simulink model "HVDC_VSC_1CPUcore_dcpl"  (Simulink 8.4)
settings: Solver=ode3  SolverMode=SingleTasking  StartTime=0.0  StopTime=70.0  FixedStep=Ts_Power  RelTol=1e-3  AbsTol=1e-2
PreLoadFcn:
  | Ts_Power=50e-6; Ts_Control=1*Ts_Power; init_cosim_IA; startup_transients_hvdc_vsc;
PostLoadFcn:
  | Ts_Power=50e-6; Ts_Control=1*Ts_Power; init_cosim_IA; startup_transients_hvdc_vsc;
InitFcn:
  | Ts_Power=50e-6; Ts_Control=1*Ts_Power; init_cosim_IA; startup_transients_hvdc_vsc;
undefined symbols (not defined in the file): CLARK, D1, Delta, dPref1_2, dPref1_2_rlimit, gcbh, h, intfDelay, level, lib_mesures, magnitude, ResistanceM, rte_drive_private_lib, rte_tsb3level_hiz_rect_cb, sps_rtmsupport, t_deblock_Pref1, t_deblock_Udref2, t_dPref1_2, t_SwitchITMIdc, t_SwitchITMVdc, Ts_intf, TSB3_hiZR
libraries: powerlib x183, spsVIMeasurementModel x102, powerlib_extras x71, powerlib_meascontrol x50, rteventslib x26, op_dpl_lib x20, rtlab x14, sps_avr x6, artemis x1
(part 10 of 13)

== system HVDC_VSC_1CPUcore_dcpl/SS_HVDCStation2_WSCC2/WSCC System 2/Bus_9 230 KV/Three-Phase V-I Measurement3 ==
  Kv : Gain  Gain=Ki  SaturateOnIntegerOverflow=on  OutDataTypeStr=Inherit: Same as input  ParamDataTypeStr=Inherit: Same as input
  Kv1 : Gain  Gain=Kv  SaturateOnIntegerOverflow=on  OutDataTypeStr=Inherit: Same as input  ParamDataTypeStr=Inherit: Same as input
  Mode I : spsVIMeasurementModel/Complex
  Mode V : spsVIMeasurementModel/Complex
  Model : spsVIMeasurementModel/VI_phase  SystemSampleTime=-1
  A : PMIOPort  Port=1  Side=Left
  B : PMIOPort  Port=2  Side=Left
  C : PMIOPort  Port=3  Side=Left
  a : PMIOPort  Port=4  Side=Right
  b : PMIOPort  Port=5  Side=Right
  c : PMIOPort  Port=6  Side=Right
  tag scope: Iabc_30=global, Vabc_30=global
  wires:
  Model/2 -> Kv/1
  Model/1 -> Kv1/1
  Kv/1 -> Mode I/1
  Kv1/1 -> Mode V/1
  Mode I/1 -> [Iabc_30]
  Mode V/1 -> [Vabc_30]
  connections:
  Model/RConn3 -- c/RConn1
  Model/RConn1 -- a/RConn1
  Model/RConn2 -- b/RConn1
  Model/LConn3 -- C/RConn1
  Model/LConn1 -- A/RConn1
  Model/LConn2 -- B/RConn1

== system HVDC_VSC_1CPUcore_dcpl/SS_HVDCStation2_WSCC2/WSCC System 2/Generator BUS1x1/Subsystem1 ==
  In1 : Inport
  In2 : Inport  Port=2
  In3 : Inport  Port=3
  Gain : Gain  Gain=-1  SaturateOnIntegerOverflow=on  OutDataTypeStr=Inherit: Same as input  ParamDataTypeStr=Inherit: Same as input
  Mux : Mux  Inputs=2
  Selector : Selector  InputPortWidth=4  Indices=[4 3]
  Selector1 : Selector  InputPortWidth=4  Indices=[4 3]
  dw_123 : Outport
  T_23 : Outport  Port=2
  wires:
  Selector/1 -> Mux/2
  Mux/1 -> dw_123/1
  In1/1 -> Mux/1
  In2/1 -> Selector/1
  In3/1 -> Selector1/1
  Selector1/1 -> Gain/1
  Gain/1 -> T_23/1

== system HVDC_VSC_1CPUcore_dcpl/SS_HVDCStation2_WSCC2/WSCC System 2/Generator BUS2x1/Subsystem1 ==
  In1 : Inport
  In2 : Inport  Port=2
  In3 : Inport  Port=3
  Gain : Gain  Gain=-1  SaturateOnIntegerOverflow=on  OutDataTypeStr=Inherit: Same as input  ParamDataTypeStr=Inherit: Same as input
  Mux : Mux  Inputs=2
  Selector : Selector  InputPortWidth=4  Indices=[4 3]
  Selector1 : Selector  InputPortWidth=4  Indices=[4 3]
  dw_123 : Outport
  T_23 : Outport  Port=2
  wires:
  Selector/1 -> Mux/2
  Mux/1 -> dw_123/1
  In1/1 -> Mux/1
  In2/1 -> Selector/1
  In3/1 -> Selector1/1
  Selector1/1 -> Gain/1
  Gain/1 -> T_23/1

== system HVDC_VSC_1CPUcore_dcpl/SS_HVDCStation2_WSCC2/WSCC System 2/Generator BUS3x1/Subsystem1 ==
  In1 : Inport
  In2 : Inport  Port=2
  In3 : Inport  Port=3
  Gain : Gain  Gain=-1  SaturateOnIntegerOverflow=on  OutDataTypeStr=Inherit: Same as input  ParamDataTypeStr=Inherit: Same as input
  Mux : Mux  Inputs=2
  Selector : Selector  InputPortWidth=4  Indices=[4 3]
  Selector1 : Selector  InputPortWidth=4  Indices=[4 3]
  dw_123 : Outport
  T_23 : Outport  Port=2
  wires:
  Selector/1 -> Mux/2
  Mux/1 -> dw_123/1
  In1/1 -> Mux/1
  In2/1 -> Selector/1
  In3/1 -> Selector1/1
  Selector1/1 -> Gain/1
  Gain/1 -> T_23/1

== system HVDC_VSC_1CPUcore_dcpl/SM_WSCC1_HVDCStation1/VSC Controller (Station 1)/Discrete VSC Controller (Station 1)/Clark Transformations/CLARK  ==
  note: CLARK transformation
  abc : Inport
  Fcn1 : Fcn  Expr=1/sqrt(3)*(u[2] - u[3])
  Fcn2 : Fcn  Expr=1/3*(2*u[1] - u[2] - u[3])
  Fcn3 : Fcn  Expr=1/3*(u[1] + u[2] + u[3])
  Mux : Mux  Inputs=3
  AB0 : Outport
  wires:
  Fcn2/1 -> Mux/1
  abc/1 -> Fcn1/1, Fcn3/1, Fcn2/1
  Fcn1/1 -> Mux/2
  Fcn3/1 -> Mux/3
  Mux/1 -> AB0/1

== system HVDC_VSC_1CPUcore_dcpl/SM_WSCC1_HVDCStation1/VSC Controller (Station 1)/Discrete VSC Controller (Station 1)/Clark Transformations/CLARK   ==
  note: CLARK transformation
  abc : Inport
  Fcn1 : Fcn  Expr=1/sqrt(3)*(u[2] - u[3])
  Fcn2 : Fcn  Expr=1/3*(2*u[1] - u[2] - u[3])
  Fcn3 : Fcn  Expr=1/3*(u[1] + u[2] + u[3])
  Mux : Mux  Inputs=3
  AB0 : Outport
  wires:
  Mux/1 -> AB0/1
  Fcn3/1 -> Mux/3
  Fcn1/1 -> Mux/2
  abc/1 -> Fcn2/1, Fcn3/1, Fcn1/1
  Fcn2/1 -> Mux/1

== system HVDC_VSC_1CPUcore_dcpl/SM_WSCC1_HVDCStation1/VSC Controller (Station 1)/Discrete VSC Controller (Station 1)/Clark Transformations/CLARK_YD ==
  note: Rotation of pi/6
  note: Rotation of - pi/6
  note: Transformer Connexion:
      | YY = 0
      | YD1 (laging) = 1
      | YD11 (leading)= 2
  note: CLARK transformation
  abc : Inport
  Tr_conx : Inport  Port=2
  CLARK : Subsystem  AncestorBlock=lib_mesures/CLARK  TreatAsAtomicUnit=on
  CLARK_YD1 : Subsystem  AncestorBlock=lib_mesures/CLARK  TreatAsAtomicUnit=on
  CLARK_YD11 : Subsystem  AncestorBlock=lib_mesures/CLARK  TreatAsAtomicUnit=on
  Constant : Constant  Value=2
  Constant1 : Constant  Value=0
  Constant2 : Constant
  Relational Operator1 : RelationalOperator  Operator===  InputSameDT=on
  Relational Operator2 : RelationalOperator  Operator===  InputSameDT=on
  Relational Operator3 : RelationalOperator  Operator===  InputSameDT=on
  Sum : Sum  Inputs=+++  SaturateOnIntegerOverflow=on
  AB0 : Outport
  wires:
  Constant2/1 -> Relational Operator3/2
  Relational Operator2/1 -> CLARK/Enable
  Constant1/1 -> Relational Operator2/2
  CLARK/1(AB0) -> Sum/3
  Sum/1 -> AB0/1
  CLARK_YD1/1(AB0) -> Sum/2
  CLARK_YD11/1(AB0) -> Sum/1
  abc/1 -> CLARK/1(abc), CLARK_YD1/1(abc), CLARK_YD11/1(abc)
  Relational Operator1/1 -> CLARK_YD11/Enable
  Relational Operator3/1 -> CLARK_YD1/Enable
  Tr_conx/1 -> Relational Operator3/1, Relational Operator2/1, Relational Operator1/1
  Constant/1 -> Relational Operator1/2

== system HVDC_VSC_1CPUcore_dcpl/SM_WSCC1_HVDCStation1/VSC Controller (Station 1)/Discrete VSC Controller (Station 1)/Clark Transformations/CLARK_YD  ==
  note: CLARK transformation
  note: Transformer Connexion:
      | YY = 0
      | YD1 (laging) = 1
      | YD11 (leading)= 2
  note: Rotation of - pi/6
  note: Rotation of pi/6
  abc : Inport
  Tr_conx : Inport  Port=2
  CLARK : Subsystem  AncestorBlock=lib_mesures/CLARK  TreatAsAtomicUnit=on
  CLARK_YD1 : Subsystem  AncestorBlock=lib_mesures/CLARK  TreatAsAtomicUnit=on
  CLARK_YD11 : Subsystem  AncestorBlock=lib_mesures/CLARK  TreatAsAtomicUnit=on
  Constant : Constant  Value=2
  Constant1 : Constant  Value=0
  Constant2 : Constant
  Relational Operator1 : RelationalOperator  Operator===  InputSameDT=on
  Relational Operator2 : RelationalOperator  Operator===  InputSameDT=on
  Relational Operator3 : RelationalOperator  Operator===  InputSameDT=on
  Sum : Sum  Inputs=+++  SaturateOnIntegerOverflow=on
  AB0 : Outport
  wires:
  Constant/1 -> Relational Operator1/2
  Tr_conx/1 -> Relational Operator1/1, Relational Operator2/1, Relational Operator3/1
  Relational Operator3/1 -> CLARK_YD1/Enable
  Relational Operator1/1 -> CLARK_YD11/Enable
  abc/1 -> CLARK_YD11/1(abc), CLARK_YD1/1(abc), CLARK/1(abc)
  CLARK_YD11/1(AB0) -> Sum/1
  CLARK_YD1/1(AB0) -> Sum/2
  Sum/1 -> AB0/1
  CLARK/1(AB0) -> Sum/3
  Constant1/1 -> Relational Operator2/2
  Relational Operator2/1 -> CLARK/Enable
  Constant2/1 -> Relational Operator3/2

== system HVDC_VSC_1CPUcore_dcpl/SM_WSCC1_HVDCStation1/VSC Controller (Station 1)/Discrete VSC Controller (Station 1)/DC Voltage Balance Control/Regulator ==
  note: Reset states when enabling
  note: Voltage Sign
  note: Reversed Current Sign
  V_ref_lim_abc : Inport
  Iv_abc : Inport  Port=2
  Udc_0_mean : Inport  Port=3
  Enable : EnablePort  StatesWhenEnabling=reset
  Constant1 : Constant  Value=0
  Constant13 : Constant  Value=Ki_dcvbc
  Constant2 : Constant  Value=0
  Constant3 : Constant  Value=-1
  Constant4 : Constant
  Constant5 : Constant
  Constant6 : Constant  Value=-1
  Constant7 : Constant  Value=0
  Constant8 : Constant  Value=Kp_dcvbc
  "PI_regulator " : Subsystem  mask(PI regulator - type 2){max_i=max_out_dcvbc, min_i=min_out_dcvbc, i_ic=0, max_out=max_out_dcvbc, min_out=min_out_dcvbc, Ts=Ts_Control}
      mask prompts: max_i "Integrator maximum  limit:"; min_i "Integrator minimum  limit:"; i_ic "Integrator initial condition:"; max_out "Output maximum limit:"; min_out "Output minimum limit:"; Ts "Sample time: (s)"
  Product : Product  Inputs=3  SaturateOnIntegerOverflow=on  OutDataTypeStr=Inherit: Same as first input
  Relational Operator : RelationalOperator  Operator=<
  Relational Operator1 : RelationalOperator  Operator=<
  Switch : Switch  Threshold=0.5  SaturateOnIntegerOverflow=on
  Switch1 : Switch  Threshold=0.5  SaturateOnIntegerOverflow=on
  dV_ref_abc_dcvbc : Outport
  wires:
  Switch1/1 -> Product/2
  Constant1/1 -> "PI_regulator "/5(Kf), "PI_regulator "/2(Meas)
  Constant13/1 -> "PI_regulator "/3(Ki)
  Constant8/1 -> "PI_regulator "/4(Kp)
  "PI_regulator "/1(Out) -> Product/3
  Constant2/1 -> Relational Operator/2
  Constant3/1 -> Switch/1
  Constant4/1 -> Switch/3
  Relational Operator/1 -> Switch/2
  Constant5/1 -> Switch1/1
  Constant6/1 -> Switch1/3
  Relational Operator1/1 -> Switch1/2
  Switch/1 -> Product/1
  V_ref_lim_abc/1 -> Relational Operator/1
  Product/1 -> dV_ref_abc_dcvbc/1
  Iv_abc/1 -> Relational Operator1/1
  Udc_0_mean/1 -> "PI_regulator "/1(Ord)
  Constant7/1 -> Relational Operator1/2

== system HVDC_VSC_1CPUcore_dcpl/SM_WSCC1_HVDCStation1/VSC Controller (Station 1)/Discrete VSC Controller (Station 1)/Inner Current Loop/AC_Current_Control ==
  note: Uq
  note: Ud
  note: AC Current Control
  note: d axis
  note: q axis
  Iv_dq : Inport
  Iref_dq : Inport  Port=2
  U_dq : Inport  Port=3
  Freq : Inport  Port=4
  Constant1 : Constant  Value=Kp_accc
  Constant13 : Constant  Value=Ki_accc
  Constant2 : Constant  Value=1.0
  Constant3 : Constant  Value=Kf_accc
  Demux : Demux  Outputs=2
  Demux1 : Demux  Outputs=2
  Demux2 : Demux  Outputs=2
  IC: 1.0 : powerlib_extras/Discrete Measurements/Discrete Variable Frequency Mean value  Finit=60  Fmin=f_min_pll  Vinit=1.0  Ts=Ts_Control
  Mux : Mux  Inputs=2
  "PI_regulator " : Subsystem  mask(PI regulator - type 2){max_i=max_out_accc, min_i=min_out_accc, i_ic=0, max_out=max_out_accc, min_out=min_out_accc, Ts=Ts_Control}
      mask prompts: max_i "Integrator maximum  limit:"; min_i "Integrator minimum  limit:"; i_ic "Integrator initial condition:"; max_out "Output maximum limit:"; min_out "Output minimum limit:"; Ts "Sample time: (s)"
  PI_regulator_2 : Subsystem  mask(PI regulator - type 2){max_i=max_out_accc, min_i=min_out_accc, i_ic=0, max_out=max_out_accc, min_out=min_out_accc, Ts=Ts_Control}
      mask prompts: max_i "Integrator maximum  limit:"; min_i "Integrator minimum  limit:"; i_ic "Integrator initial condition:"; max_out "Output maximum limit:"; min_out "Output minimum limit:"; Ts "Sample time: (s)"
  Product : Product  SaturateOnIntegerOverflow=on  OutDataTypeStr=Inherit: Same as first input
  Product1 : Product  SaturateOnIntegerOverflow=on  OutDataTypeStr=Inherit: Same as first input
  Sum2 : Sum  Inputs=+|-|+  SaturateOnIntegerOverflow=on  InputSameDT=on  OutDataTypeStr=Inherit: Same as first input
  Sum3 : Sum  Inputs=--+  SaturateOnIntegerOverflow=on  InputSameDT=on  OutDataTypeStr=Inherit: Same as first input
  "Variable Frequency Mean value IC:1.0 " : powerlib_extras/Discrete Measurements/Discrete Variable Frequency Mean value  Finit=60  Fmin=f_min_pll  Vinit=1.0  Ts=Ts_Control
  Vref_dq_tmp : Outport
  wires:
  Constant3/1 -> Product1/1, Product/2
  Sum3/1 -> Mux/2
  IC: 1.0/1 -> Sum3/3
  Demux2/2 -> IC: 1.0/2
  Product1/1 -> Sum3/2
  Sum2/1 -> Mux/1
  "Variable Frequency Mean value IC:1.0 "/1 -> Sum2/1
  Freq/1 -> IC: 1.0/1, "Variable Frequency Mean value IC:1.0 "/1
  Demux2/1 -> "Variable Frequency Mean value IC:1.0 "/2
  Product/1 -> Sum2/3
  PI_regulator_2/1(Out) -> Sum3/1
  "PI_regulator "/1(Out) -> Sum2/2
  Iref_dq/1 -> Demux1/1
  Iv_dq/1 -> Demux/1
  Demux1/1 -> "PI_regulator "/1(Ord)  "I_ref_d"
  Demux/1 -> Product1/2, "PI_regulator "/2(Meas)  "Iv_d"
  Constant2/1 -> "PI_regulator "/5(Kf), PI_regulator_2/5(Kf)
  Demux/2 -> Product/1, PI_regulator_2/2(Meas)  "Iv_q"
  Constant13/1 -> "PI_regulator "/3(Ki), PI_regulator_2/3(Ki)
  Mux/1 -> Vref_dq_tmp/1
  Constant1/1 -> "PI_regulator "/4(Kp), PI_regulator_2/4(Kp)
  Demux1/2 -> PI_regulator_2/1(Ord)  "I_ref_q"
  U_dq/1 -> Demux2/1

== system HVDC_VSC_1CPUcore_dcpl/SM_WSCC1_HVDCStation1/VSC Controller (Station 1)/Discrete VSC Controller (Station 1)/Inner Current Loop/Inverse_Clark ==
  note: Inverse CLARK transformation
  AB0 : Inport
  Fcn1 : Fcn  Expr="1/2*(-u[1]  + sqrt(3)*u[2] + 2*u[3])"
  Fcn2 : Fcn  Expr=(u[1] - u[3])
  Fcn3 : Fcn  Expr=1/2*(-u[1] - sqrt(3)*u[2] + 2*u[3])
  Mux : Mux  Inputs=3
  abc : Outport
  wires:
  Fcn2/1 -> Mux/1
  AB0/1 -> Fcn1/1, Fcn3/1, Fcn2/1
  Fcn1/1 -> Mux/2
  Fcn3/1 -> Mux/3
  Mux/1 -> abc/1

== system HVDC_VSC_1CPUcore_dcpl/SM_WSCC1_HVDCStation1/VSC Controller (Station 1)/Discrete VSC Controller (Station 1)/Inner Current Loop/Reference_Voltage_Conditioning ==
  note: Maximum AC Voltage / DC Voltage (pole-neutral)
  note: Voltage Reference Conditioning
  Vref_dq_tmp : Inport
  Udc_meas_mean : Inport  Port=2
  Constant2 : Constant  Value=K_pwm
  Gain1 : Gain  Gain=k_pu2nom_Vdc  SaturateOnIntegerOverflow=on  OutDataTypeStr=Inherit: Same as input  ParamDataTypeStr=Inherit: Same as input
  Product1 : Product  Inputs=**/  SaturateOnIntegerOverflow=on  OutDataTypeStr=Inherit: Same as first input
  Vref_dq : Outport
  wires:
  Gain1/1 -> Product1/2
  Udc_meas_mean/1 -> Gain1/1
  Product1/1 -> Vref_dq/1
  Vref_dq_tmp/1 -> Product1/1
  Constant2/1 -> Product1/3

== system HVDC_VSC_1CPUcore_dcpl/SM_WSCC1_HVDCStation1/VSC Controller (Station 1)/Discrete VSC Controller (Station 1)/Inner Current Loop/Reference_Voltage_Limitation ==
  note: Limitation on a circle of 1 p.u. radius
  note: Reference Voltage Limitation
  note: Not Limited
  note: Limited
  Vref_dq : Inport
  Constant2 : Constant  Value=1.0
  Math Function : Math  Operator=magnitude^2  SaturateOnIntegerOverflow=on
  Math Function1 : Math  Operator=sqrt  SaturateOnIntegerOverflow=on
  Max=inf Min=eps : Saturate  UpperLimit=1e6  LowerLimit=1e-6
  Product : Product  Inputs=/*  SaturateOnIntegerOverflow=on  OutDataTypeStr=Inherit: Same as first input
  Relational Operator1 : RelationalOperator  Operator=<
  Sum : Sum  Inputs=+  SaturateOnIntegerOverflow=on
  Switch : Switch  Threshold=0.5  SaturateOnIntegerOverflow=on
  Vref_lim_dq : Outport
  wires:
  Max=inf Min=eps/1 -> Product/1
  Relational Operator1/1 -> Switch/2
  Math Function1/1 -> Max=inf Min=eps/1, Relational Operator1/1
  Vref_dq/1 -> Math Function/1, Switch/1, Product/2
  Math Function/1 -> Sum/1
  Sum/1 -> Math Function1/1
  Product/1 -> Switch/3
  Switch/1 -> Vref_lim_dq/1
  Constant2/1 -> Relational Operator1/2

== system HVDC_VSC_1CPUcore_dcpl/SM_WSCC1_HVDCStation1/VSC Controller (Station 1)/Discrete VSC Controller (Station 1)/Inner Current Loop/dq0 to abo ==
  note: X0 = X0
  note: dq0 to ab0
  note: Xa = Xd*sin(wt) + Xq*cos(wt)
  note: Xb = -Xd*cos(wt) + Xq*sin(wt)
  dq0 : Inport
  sin_cos : Inport  Port=2
  Demux : Demux  Outputs=2
  Demux1 : Demux  Outputs=3
  Mux : Mux  Inputs=3
  Product{,1..3} (4 alike) : Product  SaturateOnIntegerOverflow=on  InputSameDT=on  OutDataTypeStr=Inherit: Same as first input
  Sum1 : Sum  Inputs=+-  SaturateOnIntegerOverflow=on  InputSameDT=on  OutDataTypeStr=Inherit: Same as first input
  Sum4 : Sum  Inputs=2  SaturateOnIntegerOverflow=on  InputSameDT=on  OutDataTypeStr=Inherit: Same as first input
  ab0 : Outport
  wires:
  dq0/1 -> Demux1/1
  Mux/1 -> ab0/1
  Product3/1 -> Sum1/2
  Product2/1 -> Sum1/1
  Product1/1 -> Sum4/1
  Product/1 -> Sum4/2
  sin_cos/1 -> Demux/1
  Sum4/1 -> Mux/1
  Demux1/1 -> Product1/1, Product3/1
  Demux/1 -> Product1/2, Product2/2
  Demux/2 -> Product/2, Product3/2
  Demux1/2 -> Product/1, Product2/1
  Sum1/1 -> Mux/2
  Demux1/3 -> Mux/3

== system HVDC_VSC_1CPUcore_dcpl/SM_WSCC1_HVDCStation1/VSC Controller (Station 1)/Discrete VSC Controller (Station 1)/Outer Active-Reactive Power and Voltage Loop/Active_Power_Control ==
  note: Active Power Control
  enable_control : Inport
  enable_ramp : Inport  Port=2
  Pref : Inport  Port=3
  dPref : Inport  Port=4
  P_meas : Inport  Port=5
  U_meas : Inport  Port=6
  Udc_meas : Inport  Port=7
  Constant1 : Constant  Value=Udc_max
  Constant11 : Constant  Value=Ki_apc
  Constant12 : Constant  Value=Ramp_apc
  Constant13 : Constant  Value=P_max
  Constant14 : Constant  Value=P_min
  Constant2 : Constant  Value=Udc_min
  Constant25 : Constant  Value=Ki_apc_vco
  Constant3 : Constant  Value=Kp_apc_vco
  DC Voltage Control Override : Subsystem  TreatAsAtomicUnit=on
  Freeze_integrator : Subsystem
  Max=P_max Min=P_min : Saturate  UpperLimit=P_max  LowerLimit=P_min
  Ramping : Subsystem
  Regulator : Subsystem  TreatAsAtomicUnit=on
  Sum1 : Sum  SaturateOnIntegerOverflow=on
  Sum2 : Sum  SaturateOnIntegerOverflow=on
  Pref_apc : Outport
  Pref_ramped : Outport  Port=2
  wires:
  U_meas/1 -> Freeze_integrator/1(U_meas)
  Freeze_integrator/1(Freeze) -> Regulator/6(Freeze)
  Constant14/1 -> Regulator/5(min_out)
  Constant13/1 -> Regulator/4(max_out)
  enable_ramp/1 -> Ramping/1(enable_ramp)
  Pref/1 -> Ramping/2(Pref)
  Constant12/1 -> Ramping/3(ramp_apc)
  P_meas/1 -> Regulator/2(Meas)
  Constant11/1 -> Regulator/3(Ki)
  Sum2/1 -> Regulator/1(Ord), Pref_ramped/1
  dPref/1 -> Sum2/2
  Ramping/1(Pref_ramp) -> Sum2/1
  enable_control/1 -> Regulator/Enable, DC Voltage Control Override/Enable
  Regulator/1(Out) -> Sum1/1
  Sum1/1 -> Max=P_max Min=P_min/1
  DC Voltage Control Override/1(Out) -> Sum1/2
  Constant25/1 -> DC Voltage Control Override/1(Ki_apc_vco)
  Constant1/1 -> DC Voltage Control Override/3(Udc_max)
  Constant2/1 -> DC Voltage Control Override/4(Udc_min)
  Udc_meas/1 -> DC Voltage Control Override/5(Udc_meas)
  Constant3/1 -> DC Voltage Control Override/2(Kp_apc_vco)
  Max=P_max Min=P_min/1 -> Pref_apc/1

== system HVDC_VSC_1CPUcore_dcpl/SM_WSCC1_HVDCStation1/VSC Controller (Station 1)/Discrete VSC Controller (Station 1)/Outer Active-Reactive Power and Voltage Loop/Current_Reference_Calculation ==
  note: Current Reference Calculation
  Pref_apc : Inport
  Qref_rpc : Inport  Port=2
  Uf_meas : Inport  Port=3
  2nd-Order Filter : powerlib_extras/Discrete  Control Blocks/Discrete  2nd-Order Filter  FilterType=Lowpass  Fo=f0_crc  Zeta=1/sqrt(2)  Ts=Ts_Control  Initialize=off  Vac_Init=[0.8 -25 60]  Vdc_Init=-0.4  PlotResponse=off  param1=[1 500 1]
  Constant22 : Constant  Value=lim_d_crc
  Constant23 : Constant  Value=lim_q_crc
  Constant24 : Constant  Value=U_level_crc
  Gain1 : Gain  Gain=-1  SaturateOnIntegerOverflow=on  OutDataTypeStr=Inherit: Same as input  ParamDataTypeStr=Inherit: Same as input
  Gain2 : Gain  Gain=-1  SaturateOnIntegerOverflow=on  OutDataTypeStr=Inherit: Same as input  ParamDataTypeStr=Inherit: Same as input
  MinMax : MinMax  Function=max  Inputs=2  SaturateOnIntegerOverflow=on  InputSameDT=on
  Product : Product  Inputs=*/  SaturateOnIntegerOverflow=on  OutDataTypeStr=Inherit: Same as first input
  Product1 : Product  Inputs=/*  SaturateOnIntegerOverflow=on  OutDataTypeStr=Inherit: Same as first input
  S1 : Subsystem  AncestorBlock=|  mask(Limiter with External Limits){}
      | powerlib_extras/Discrete 
      | Control Blocks/Discrete 12-Pulse
      | HVDC Control /Functions
      | (Discrete)/Current Regulator/S16/S6
      mask Display: disp('      Limiter\n')
  S2 : Subsystem  AncestorBlock=|  mask(Limiter with External Limits){}
      | powerlib_extras/Discrete 
      | Control Blocks/Discrete 12-Pulse
      | HVDC Control /Functions
      | (Discrete)/Current Regulator/S16/S6
      mask Display: disp('      Limiter\n')
  sat : Saturate  UpperLimit=1e6  LowerLimit=1e-6
  Iref_d_crc : Outport
  Iref_q_crc : Outport  Port=2
  wires:
  2nd-Order Filter/1 -> MinMax/2
  S2/1("  ") -> Iref_q_crc/1
  S1/1("  ") -> Iref_d_crc/1
  Uf_meas/1 -> 2nd-Order Filter/1
  Constant24/1 -> MinMax/1
  Pref_apc/1 -> Product/1
  sat/1 -> Product/2, Product1/1
  Qref_rpc/1 -> Product1/2
  Product/1 -> S1/2(In)
  Product1/1 -> S2/2(In)
  Constant22/1 -> Gain1/1, S1/1(MAX)
  Gain1/1 -> S1/3(MIN)
  Constant23/1 -> Gain2/1, S2/1(MAX)
  Gain2/1 -> S2/3(MIN)
  MinMax/1 -> sat/1

== system HVDC_VSC_1CPUcore_dcpl/SM_WSCC1_HVDCStation1/VSC Controller (Station 1)/Discrete VSC Controller (Station 1)/Outer Active-Reactive Power and Voltage Loop/Current_Reference_Limitation ==
  note: DC Voltage Control mode (Active power priority)
  note: Power Control mode (Equal scaling)
  note: Current Reference Limitation
  Iref_d_tmp : Inport  PortDimensions=1
  Iref_q_tmp : Inport  Port=2  PortDimensions=1
  P_control : Inport  Port=3
  Constant25 : Constant  Value=Iref_max
  Double click here for  info : Subsystem
      mask Display: disp('?')
  Math Function1 : Math  Operator=sqrt  SaturateOnIntegerOverflow=on
  Math Function2 : Math  Operator=magnitude^2  SaturateOnIntegerOverflow=on
  Math Function3 : Math  Operator=magnitude^2  SaturateOnIntegerOverflow=on
  Math Function4 : Math  Operator=magnitude^2  SaturateOnIntegerOverflow=on
  Math Function5 : Math  Operator=sqrt  SaturateOnIntegerOverflow=on
  Min:eps Max:inf : Saturate  UpperLimit=1e6  LowerLimit=1e-6
  Mux : Mux  Inputs=2
  Mux1 : Mux  Inputs=2
  Product1 : Product  SaturateOnIntegerOverflow=on  OutDataTypeStr=Inherit: Same as first input
  Product2 : Product  Inputs=*/  SaturateOnIntegerOverflow=on  OutDataTypeStr=Inherit: Same as first input
  Relational Operator1 : RelationalOperator
  Relational Operator3 : RelationalOperator
  Sign : Signum
  Sum : Sum  Inputs=+  SaturateOnIntegerOverflow=on
  Sum2 : Sum  Inputs=-+  SaturateOnIntegerOverflow=on
  Switch1 : Switch  Threshold=0.5  SaturateOnIntegerOverflow=on
  Switch2 : Switch  Threshold=0.5  SaturateOnIntegerOverflow=on
  Switch3 : Switch  Threshold=0.5  SaturateOnIntegerOverflow=on
  Iref_dq : Outport
  wires:
  Sign/1 -> Product1/2
  Math Function5/1 -> Product1/1
  Product1/1 -> Mux1/2
  Sum2/1 -> Math Function5/1
  Math Function4/1 -> Sum2/1
  Math Function3/1 -> Sum2/2
  Mux1/1 -> Switch2/3
  Switch1/1 -> Iref_dq/1
  Switch2/1 -> Switch1/1
  Product2/1 -> Switch2/1
  Min:eps Max:inf/1 -> Product2/2
  Relational Operator1/1 -> Switch1/2
  Constant25/1 -> Relational Operator3/2, Switch3/1, Math Function3/1, Relational Operator1/2
  Math Function1/1 -> Min:eps Max:inf/1, Relational Operator1/1
  Mux/1 -> Product2/1, Math Function2/1, Switch1/3
  Iref_q_tmp/1 -> Sign/1, Mux/2
  Iref_d_tmp/1 -> Relational Operator3/1, Switch3/3, Mux/1
  Sum/1 -> Math Function1/1
  Math Function2/1 -> Sum/1
  P_control/1 -> Switch2/2
  Relational Operator3/1 -> Switch3/2
  Switch3/1 -> Mux1/1, Math Function4/1

== system HVDC_VSC_1CPUcore_dcpl/SM_WSCC1_HVDCStation1/VSC Controller (Station 1)/Discrete VSC Controller (Station 1)/Outer Active-Reactive Power and Voltage Loop/DC_Voltage_Control ==
  note: DC Voltage Control
  note: Reset integrator when enabling
  note: pu DC --> pu AC
  Udref : Inport
  Udc_meas : Inport  Port=2
  Ki_dcvc : Inport  Port=3
  Kp_dcvc : Inport  Port=4
  Enable : EnablePort  StatesWhenEnabling=reset
  Constant1 : Constant  Value=0
  Constant2 : Constant  Value=max_i_dcvc
  Constant3 : Constant  Value=min_i_dcvc
  Constant4 : Constant  Value=max_out_dcvc
  Constant5 : Constant
  Constant6 : Constant  Value=min_out_dcvc
  First-Order_LP f0_Udc IC= k_nom2pu_Vdc : powerlib_extras/Discrete  Control Blocks/Discrete 1st-Order Filter  FilterType=Lowpass  Tc=1/(2*pi*f0_Udc)  Ts=Ts_Control  Initialize=on  Vac_Init=[0 0 60]  Vdc_Init=k_nom2pu_Vdc  PlotResponse=off  param1=[1 600 0.1]
  Gain1 : Gain  Gain=k_nom2pu_Vdc  SaturateOnIntegerOverflow=on  OutDataTypeStr=Inherit: Same as input  ParamDataTypeStr=Inherit: Same as input
  Ic=0 : UnitDelay  SampleTime=Ts_Control
  Kf_dcvc : Constant  Value=1.0
  Logical Operator : Logic  Operator=NOT  Inputs=1  AllPortsSameDT=off
  PI : Subsystem  mask(Integrator  With  External  Dynamic  Limits (Discrete)){i_ic=0, Ts=Ts_Control}
      mask prompts: i_ic "Initial Condition:"; Ts "Sample time: (s)"
      mask Display: disp('Discrete-Time\n(Trapezoidal)\nIntegrator\n ')
  Product2 : Product  SaturateOnIntegerOverflow=on  OutDataTypeStr=Inherit: Same as first input
  Product3 : Product  SaturateOnIntegerOverflow=on  OutDataTypeStr=Inherit: Same as first input
  S6 : Subsystem  AncestorBlock=|  mask(Limiter with External Limits){}
      | powerlib_extras/Discrete 
      | Control Blocks/Discrete 12-Pulse
      | HVDC Control /Functions
      | (Discrete)/Current Regulator/S16/S6
      mask Display: disp('      Limiter\n')
  Sum1 : Sum  Inputs=+-  SaturateOnIntegerOverflow=on
  Sum2 : Sum  SaturateOnIntegerOverflow=on
  Sum3 : Sum  Inputs=|+-  SaturateOnIntegerOverflow=on
  Sum4 : Sum  SaturateOnIntegerOverflow=on
  Iref_d_dcvc : Outport
  wires:
  Product3/1 -> Sum2/1
  Kp_dcvc/1 -> Product3/1
  Logical Operator/1 -> PI/5(Hold), PI/6(Reset)
  Constant5/1 -> Logical Operator/1
  Constant1/1 -> PI/7(Reset Value)
  Constant3/1 -> PI/2(Min)
  Constant2/1 -> PI/1(Max)
  Constant6/1 -> S6/3(MIN)
  Constant4/1 -> S6/1(MAX)
  Sum2/1 -> S6/2(In), Sum3/2
  Sum1/1 -> Product3/2, Sum4/1
  PI/1(Out) -> Sum2/2
  Udc_meas/1 -> First-Order_LP f0_Udc IC= k_nom2pu_Vdc/1
  Ki_dcvc/1 -> PI/4(Ki)
  S6/1("  ") -> Sum3/1, Iref_d_dcvc/1
  Sum4/1 -> PI/3(In)
  Ic=0/1 -> Sum4/2
  Sum3/1 -> Product2/2
  Product2/1 -> Ic=0/1
  Kf_dcvc/1 -> Product2/1
  First-Order_LP f0_Udc IC= k_nom2pu_Vdc/1 -> Sum1/2
  Udref/1 -> Gain1/1
  Gain1/1 -> Sum1/1

== system HVDC_VSC_1CPUcore_dcpl/SM_WSCC1_HVDCStation1/VSC Controller (Station 1)/Discrete VSC Controller (Station 1)/Outer Active-Reactive Power and Voltage Loop/Reactive_Power_Control ==
  note: Reactive Power Control
  enable_control : Inport
  Qref : Inport  Port=2
  Q_meas : Inport  Port=3
  U_meas : Inport  Port=4
  AC Voltage Control Override : Subsystem  TreatAsAtomicUnit=on
  Constant1 : Constant  Value=U_max
  Constant2 : Constant  Value=U_min
  Constant25 : Constant  Value=Ki_rpc_vco
  Constant3 : Constant  Value=Kp_rpc_vco
  Constant4 : Constant  Value=Ki_rpc
  Constant5 : Constant  Value=Q_max
  Constant6 : Constant  Value=Q_min
  Freeze_integrator : Subsystem
  Max=Q_max Min=Q_min : Saturate  UpperLimit=Q_max  LowerLimit=Q_min
  Regulator : Subsystem  TreatAsAtomicUnit=on
  Sum2 : Sum  SaturateOnIntegerOverflow=on
  Qref_rpc : Outport
  wires:
  Sum2/1 -> Max=Q_max Min=Q_min/1
  Regulator/1(Out) -> Sum2/1
  Qref/1 -> Regulator/1(Ord)
  Constant5/1 -> Regulator/4(max_out)
  Constant6/1 -> Regulator/5(min_out)
  Constant4/1 -> Regulator/3(Ki)
  Q_meas/1 -> Regulator/2(Meas)
  U_meas/1 -> AC Voltage Control Override/5(U_meas), Freeze_integrator/1(U_meas)
  enable_control/1 -> Regulator/Enable, AC Voltage Control Override/Enable
  Constant25/1 -> AC Voltage Control Override/1(Ki_rpc_vco)
  Constant3/1 -> AC Voltage Control Override/2(Kp_rpc_vco)
  Constant1/1 -> AC Voltage Control Override/3(U_max)
  Constant2/1 -> AC Voltage Control Override/4(U_min)
  AC Voltage Control Override/1(Out) -> Sum2/2
  Max=Q_max Min=Q_min/1 -> Qref_rpc/1
  Freeze_integrator/1(Freeze) -> Regulator/6(freeze)

== system HVDC_VSC_1CPUcore_dcpl/SM_WSCC1_HVDCStation1/VSC Controller (Station 1)/Discrete VSC Controller (Station 1)/PLL/ab0->dq0  ==
  note: Xq = Xa*cos(wt) + Xb*sin(wt)
  note: Xd = Xa*sin(wt) - Xb*cos(wt)
  note: Alpha-Beta-zero to dq0
  note: X0 = X0
  ab0 : Inport
  sin_cos : Inport  Port=2
  Demux : Demux  Outputs=2
  Demux1 : Demux  Outputs=3
  Mux : Mux  Inputs=3
  Product{,1..3} (4 alike) : Product  SaturateOnIntegerOverflow=on  InputSameDT=on  OutDataTypeStr=Inherit: Same as first input
  Sum1 : Sum  Inputs=+-  SaturateOnIntegerOverflow=on  InputSameDT=on  OutDataTypeStr=Inherit: Same as first input
  Sum4 : Sum  Inputs=2  SaturateOnIntegerOverflow=on  InputSameDT=on  OutDataTypeStr=Inherit: Same as first input
  dq0 : Outport
  wires:
  Sum4/1 -> Mux/2
  Sum1/1 -> Mux/1
  sin_cos/1 -> Demux/1
  Demux/2 -> Product/2, Product3/2
  Demux1/1 -> Product/1, Product2/1
  Product/1 -> Sum4/2
  Demux/1 -> Product2/2, Product1/2
  Demux1/2 -> Product1/1, Product3/1
  Product1/1 -> Sum4/1
  Product2/1 -> Sum1/1
  Product3/1 -> Sum1/2
  Mux/1 -> dq0/1
  ab0/1 -> Demux1/1
  Demux1/3 -> Mux/3

== system HVDC_VSC_1CPUcore_dcpl/SM_WSCC1_HVDCStation1/VSC Controller (Station 1)/Discrete VSC Controller (Station 1)/Signal Calculations/Active_Power ==
  note: Active Power Calculation
  U_AB : Inport
  I_AB : Inport  Port=2
  Demux : Demux  Outputs=2
  Demux1 : Demux  Outputs=2
  Product : Product  SaturateOnIntegerOverflow=on  OutDataTypeStr=Inherit: Same as first input
  Product1 : Product  SaturateOnIntegerOverflow=on  OutDataTypeStr=Inherit: Same as first input
  Sum : Sum  SaturateOnIntegerOverflow=on
  Ppcc : Outport
  wires:
  U_AB/1 -> Demux/1
  I_AB/1 -> Demux1/1
  Demux/1 -> Product/1
  Demux1/1 -> Product/2
  Demux/2 -> Product1/1
  Demux1/2 -> Product1/2
  Product/1 -> Sum/1
  Product1/1 -> Sum/2
  Sum/1 -> Ppcc/1

== system HVDC_VSC_1CPUcore_dcpl/SM_WSCC1_HVDCStation1/VSC Controller (Station 1)/Discrete VSC Controller (Station 1)/Signal Calculations/DC_Current ==
  note: DC Current Calculation
  Idc_p : Inport
  Idc_n : Inport  Port=2
  Gain : Gain  Gain=0.5  SaturateOnIntegerOverflow=on  OutDataTypeStr=Inherit: Same as input  ParamDataTypeStr=Inherit: Same as input
  Sum : Sum  Inputs=+-  SaturateOnIntegerOverflow=on
  Idc_meas : Outport
  wires:
  Gain/1 -> Idc_meas/1
  Sum/1 -> Gain/1
  Idc_n/1 -> Sum/2
  Idc_p/1 -> Sum/1

== system HVDC_VSC_1CPUcore_dcpl/SM_WSCC1_HVDCStation1/VSC Controller (Station 1)/Discrete VSC Controller (Station 1)/Signal Calculations/DC_Voltage ==
  note: DC Voltage Calculation
  Udc_p : Inport
  Udc_n : Inport  Port=2
  Gain : Gain  Gain=0.5  SaturateOnIntegerOverflow=on  OutDataTypeStr=Inherit: Same as input  ParamDataTypeStr=Inherit: Same as input
  Sum : Sum  Inputs=+-  SaturateOnIntegerOverflow=on
  Udc_meas : Outport
  wires:
  Udc_p/1 -> Sum/1
  Sum/1 -> Gain/1
  Gain/1 -> Udc_meas/1
  Udc_n/1 -> Sum/2

== system HVDC_VSC_1CPUcore_dcpl/SM_WSCC1_HVDCStation1/VSC Controller (Station 1)/Discrete VSC Controller (Station 1)/Signal Calculations/Filter_Bus_Voltage ==
  note: Filter Bus Voltage Calculation
  Uf_AB : Inport
  Math Function : Math  Operator=magnitude^2  SaturateOnIntegerOverflow=on
  Math Function1 : Math  Operator=sqrt  SaturateOnIntegerOverflow=on
  Sum : Sum  Inputs=+  SaturateOnIntegerOverflow=on
  Uf_meas : Outport
  wires:
  Math Function1/1 -> Uf_meas/1
  Sum/1 -> Math Function1/1
  Math Function/1 -> Sum/1
  Uf_AB/1 -> Math Function/1

== system HVDC_VSC_1CPUcore_dcpl/SM_WSCC1_HVDCStation1/VSC Controller (Station 1)/Discrete VSC Controller (Station 1)/Signal Calculations/Modulation_Index ==
  note: Modulation Index Calculation
  Vref_lim_AB : Inport
  Udc_meas : Inport  Port=2
  Gain1 : Gain  Gain=k_pu2nom_Vdc  SaturateOnIntegerOverflow=on  OutDataTypeStr=Inherit: Same as input  ParamDataTypeStr=Inherit: Same as input
  MAX:10 MIN: 0 : Saturate  UpperLimit=10  LowerLimit=0
  Math Function1 : Math  Operator=magnitude^2  SaturateOnIntegerOverflow=on
  Math Function2 : Math  Operator=sqrt  SaturateOnIntegerOverflow=on
  Product : Product  Inputs=*/  SaturateOnIntegerOverflow=on  OutDataTypeStr=Inherit: Same as first input
  Saturation : Saturate  UpperLimit=1e6  LowerLimit=1e-6
  Sum : Sum  Inputs=+  SaturateOnIntegerOverflow=on
  Mod_index : Outport
  wires:
  Gain1/1 -> Saturation/1
  MAX:10 MIN: 0/1 -> Mod_index/1
  Saturation/1 -> Product/2
  Product/1 -> MAX:10 MIN: 0/1
  Udc_meas/1 -> Gain1/1
  Sum/1 -> Math Function2/1
  Math Function1/1 -> Sum/1
  Math Function2/1 -> Product/1
  Vref_lim_AB/1 -> Math Function1/1

== system HVDC_VSC_1CPUcore_dcpl/SM_WSCC1_HVDCStation1/VSC Controller (Station 1)/Discrete VSC Controller (Station 1)/Signal Calculations/PCC_Voltage ==
  note: Active Power Calculation
  U_AB : Inport
  Math Function : Math  Operator=magnitude^2  SaturateOnIntegerOverflow=on
  Math Function1 : Math  Operator=sqrt  SaturateOnIntegerOverflow=on
  Sum : Sum  Inputs=+  SaturateOnIntegerOverflow=on
  Upcc : Outport
  wires:
  U_AB/1 -> Math Function/1
  Math Function/1 -> Sum/1
  Sum/1 -> Math Function1/1
  Math Function1/1 -> Upcc/1

== system HVDC_VSC_1CPUcore_dcpl/SM_WSCC1_HVDCStation1/VSC Controller (Station 1)/Discrete VSC Controller (Station 1)/Signal Calculations/Reactive_Power ==
  note: Reactive Power Calculation
  U_AB : Inport
  I_AB : Inport  Port=2
  Demux : Demux  Outputs=2
  Demux1 : Demux  Outputs=2
  Product : Product  SaturateOnIntegerOverflow=on  OutDataTypeStr=Inherit: Same as first input
  Product1 : Product  SaturateOnIntegerOverflow=on  OutDataTypeStr=Inherit: Same as first input
  Sum : Sum  Inputs=+-  SaturateOnIntegerOverflow=on
  Qpcc : Outport
  wires:
  Sum/1 -> Qpcc/1
  Product1/1 -> Sum/2
  Product/1 -> Sum/1
  I_AB/1 -> Demux1/1
  U_AB/1 -> Demux/1
  Demux/2 -> Product/2
  Demux1/1 -> Product/1
  Demux/1 -> Product1/1
  Demux1/2 -> Product1/2

== system HVDC_VSC_1CPUcore_dcpl/SM_WSCC1_HVDCStation1/VSC Controller (Station 1)/Discrete VSC Controller (Station 1)/dq  Transformations/ab0_to_dq0 ==
  note: X0 = X0
  note: Alpha-Beta-zero to dq0
  note: Xd = Xa*sin(wt) - Xb*cos(wt)
  note: Xq = Xa*cos(wt) + Xb*sin(wt)
  ab0 : Inport
  sin_cos : Inport  Port=2
  Demux : Demux  Outputs=2
  Demux1 : Demux  Outputs=3
  Gain3 : Gain  Gain=-1  SaturateOnIntegerOverflow=on  OutDataTypeStr=Inherit: Same as input  ParamDataTypeStr=Inherit: Same as input
  Mux : Mux  Inputs=3
  Product{,1..3} (4 alike) : Product  SaturateOnIntegerOverflow=on  InputSameDT=on  OutDataTypeStr=Inherit: Same as first input
  Sum1 : Sum  Inputs=2  SaturateOnIntegerOverflow=on  InputSameDT=on  OutDataTypeStr=Inherit: Same as first input
  Sum4 : Sum  Inputs=2  SaturateOnIntegerOverflow=on  InputSameDT=on  OutDataTypeStr=Inherit: Same as first input
  dq0 : Outport
  wires:
  Demux1/3 -> Mux/3
  ab0/1 -> Demux1/1
  Mux/1 -> dq0/1
  Product3/1 -> Sum1/2
  Product2/1 -> Sum1/1
  Product1/1 -> Sum4/1
  Demux1/2 -> Product3/1, Product1/1
  Demux/1 -> Product1/2, Product2/2
  Product/1 -> Sum4/2
  Demux1/1 -> Product2/1, Product/1
  Demux/2 -> Product/2, Gain3/1
  sin_cos/1 -> Demux/1
  Sum1/1 -> Mux/1
  Gain3/1 -> Product3/2
  Sum4/1 -> Mux/2

== system HVDC_VSC_1CPUcore_dcpl/SM_WSCC1_HVDCStation1/VSC Controller (Station 1)/Discrete VSC Controller (Station 1)/dq  Transformations/ab0_to_dq0    ==
  note: Xq = Xa*cos(wt) + Xb*sin(wt)
  note: Xd = Xa*sin(wt) - Xb*cos(wt)
  note: Alpha-Beta-zero to dq0
  note: X0 = X0
  ab0 : Inport
  sin_cos : Inport  Port=2
  Demux : Demux  Outputs=2
  Demux1 : Demux  Outputs=3
  Gain3 : Gain  Gain=-1  SaturateOnIntegerOverflow=on  OutDataTypeStr=Inherit: Same as input  ParamDataTypeStr=Inherit: Same as input
  Mux : Mux  Inputs=3
  Product{,1..3} (4 alike) : Product  SaturateOnIntegerOverflow=on  InputSameDT=on  OutDataTypeStr=Inherit: Same as first input
  Sum1 : Sum  Inputs=2  SaturateOnIntegerOverflow=on  InputSameDT=on  OutDataTypeStr=Inherit: Same as first input
  Sum4 : Sum  Inputs=2  SaturateOnIntegerOverflow=on  InputSameDT=on  OutDataTypeStr=Inherit: Same as first input
  dq0 : Outport
  wires:
  Sum4/1 -> Mux/2
  Gain3/1 -> Product3/2
  Sum1/1 -> Mux/1
  sin_cos/1 -> Demux/1
  Demux/2 -> Gain3/1, Product/2
  Demux1/1 -> Product/1, Product2/1
  Product/1 -> Sum4/2
  Demux/1 -> Product2/2, Product1/2
  Demux1/2 -> Product1/1, Product3/1
  Product1/1 -> Sum4/1
  Product2/1 -> Sum1/1
  Product3/1 -> Sum1/2
  Mux/1 -> dq0/1
  ab0/1 -> Demux1/1
  Demux1/3 -> Mux/3

== system HVDC_VSC_1CPUcore_dcpl/SS_HVDCStation2_WSCC2/VSC Controller (Station 2)/Discrete VSC Controller (Station 2)/Clark Transformations/CLARK  ==
  note: CLARK transformation
  abc : Inport
  Fcn1 : Fcn  Expr=1/sqrt(3)*(u[2] - u[3])
  Fcn2 : Fcn  Expr=1/3*(2*u[1] - u[2] - u[3])
  Fcn3 : Fcn  Expr=1/3*(u[1] + u[2] + u[3])
  Mux : Mux  Inputs=3
  AB0 : Outport
  wires:
  Fcn2/1 -> Mux/1
  abc/1 -> Fcn1/1, Fcn3/1, Fcn2/1
  Fcn1/1 -> Mux/2
  Fcn3/1 -> Mux/3
  Mux/1 -> AB0/1

== system HVDC_VSC_1CPUcore_dcpl/SS_HVDCStation2_WSCC2/VSC Controller (Station 2)/Discrete VSC Controller (Station 2)/Clark Transformations/CLARK   ==
  note: CLARK transformation
  abc : Inport
  Fcn1 : Fcn  Expr=1/sqrt(3)*(u[2] - u[3])
  Fcn2 : Fcn  Expr=1/3*(2*u[1] - u[2] - u[3])
  Fcn3 : Fcn  Expr=1/3*(u[1] + u[2] + u[3])
  Mux : Mux  Inputs=3
  AB0 : Outport
  wires:
  Mux/1 -> AB0/1
  Fcn3/1 -> Mux/3
  Fcn1/1 -> Mux/2
  abc/1 -> Fcn2/1, Fcn3/1, Fcn1/1
  Fcn2/1 -> Mux/1

== system HVDC_VSC_1CPUcore_dcpl/SS_HVDCStation2_WSCC2/VSC Controller (Station 2)/Discrete VSC Controller (Station 2)/Clark Transformations/CLARK_YD ==
  note: Rotation of pi/6
  note: Rotation of - pi/6
  note: Transformer Connexion:
      | YY = 0
      | YD1 (laging) = 1
      | YD11 (leading)= 2
  note: CLARK transformation
  abc : Inport
  Tr_conx : Inport  Port=2
  CLARK : Subsystem  AncestorBlock=lib_mesures/CLARK  TreatAsAtomicUnit=on
  CLARK_YD1 : Subsystem  AncestorBlock=lib_mesures/CLARK  TreatAsAtomicUnit=on
  CLARK_YD11 : Subsystem  AncestorBlock=lib_mesures/CLARK  TreatAsAtomicUnit=on
  Constant : Constant  Value=2
  Constant1 : Constant  Value=0
  Constant2 : Constant
  Relational Operator1 : RelationalOperator  Operator===  InputSameDT=on
  Relational Operator2 : RelationalOperator  Operator===  InputSameDT=on
  Relational Operator3 : RelationalOperator  Operator===  InputSameDT=on
  Sum : Sum  Inputs=+++  SaturateOnIntegerOverflow=on
  AB0 : Outport
  wires:
  Constant2/1 -> Relational Operator3/2
  Relational Operator2/1 -> CLARK/Enable
  Constant1/1 -> Relational Operator2/2
  CLARK/1(AB0) -> Sum/3
  Sum/1 -> AB0/1
  CLARK_YD1/1(AB0) -> Sum/2
  CLARK_YD11/1(AB0) -> Sum/1
  abc/1 -> CLARK/1(abc), CLARK_YD1/1(abc), CLARK_YD11/1(abc)
  Relational Operator1/1 -> CLARK_YD11/Enable
  Relational Operator3/1 -> CLARK_YD1/Enable
  Tr_conx/1 -> Relational Operator3/1, Relational Operator2/1, Relational Operator1/1
  Constant/1 -> Relational Operator1/2

== system HVDC_VSC_1CPUcore_dcpl/SS_HVDCStation2_WSCC2/VSC Controller (Station 2)/Discrete VSC Controller (Station 2)/Clark Transformations/CLARK_YD  ==
  note: CLARK transformation
  note: Transformer Connexion:
      | YY = 0
      | YD1 (laging) = 1
      | YD11 (leading)= 2
  note: Rotation of - pi/6
  note: Rotation of pi/6
  abc : Inport
  Tr_conx : Inport  Port=2
  CLARK : Subsystem  AncestorBlock=lib_mesures/CLARK  TreatAsAtomicUnit=on
  CLARK_YD1 : Subsystem  AncestorBlock=lib_mesures/CLARK  TreatAsAtomicUnit=on
  CLARK_YD11 : Subsystem  AncestorBlock=lib_mesures/CLARK  TreatAsAtomicUnit=on
  Constant : Constant  Value=2
  Constant1 : Constant  Value=0
  Constant2 : Constant
  Relational Operator1 : RelationalOperator  Operator===  InputSameDT=on
  Relational Operator2 : RelationalOperator  Operator===  InputSameDT=on
  Relational Operator3 : RelationalOperator  Operator===  InputSameDT=on
  Sum : Sum  Inputs=+++  SaturateOnIntegerOverflow=on
  AB0 : Outport
  wires:
  Constant/1 -> Relational Operator1/2
  Tr_conx/1 -> Relational Operator1/1, Relational Operator2/1, Relational Operator3/1
  Relational Operator3/1 -> CLARK_YD1/Enable
  Relational Operator1/1 -> CLARK_YD11/Enable
  abc/1 -> CLARK_YD11/1(abc), CLARK_YD1/1(abc), CLARK/1(abc)
  CLARK_YD11/1(AB0) -> Sum/1
  CLARK_YD1/1(AB0) -> Sum/2
  Sum/1 -> AB0/1
  CLARK/1(AB0) -> Sum/3
  Constant1/1 -> Relational Operator2/2
  Relational Operator2/1 -> CLARK/Enable
  Constant2/1 -> Relational Operator3/2

== system HVDC_VSC_1CPUcore_dcpl/SS_HVDCStation2_WSCC2/VSC Controller (Station 2)/Discrete VSC Controller (Station 2)/DC Voltage Balance Control/Regulator ==
  note: Reset states when enabling
  note: Voltage Sign
  note: Reversed Current Sign
  V_ref_lim_abc : Inport
  Iv_abc : Inport  Port=2
  Udc_0_mean : Inport  Port=3
  Enable : EnablePort  StatesWhenEnabling=reset
  Constant1 : Constant  Value=0
  Constant13 : Constant  Value=Ki_dcvbc
  Constant2 : Constant  Value=0
  Constant3 : Constant  Value=-1
  Constant4 : Constant
  Constant5 : Constant
  Constant6 : Constant  Value=-1
  Constant7 : Constant  Value=0
  Constant8 : Constant  Value=Kp_dcvbc
  "PI_regulator " : Subsystem  mask(PI regulator - type 2){max_i=max_out_dcvbc, min_i=min_out_dcvbc, i_ic=0, max_out=max_out_dcvbc, min_out=min_out_dcvbc, Ts=Ts_Control}
      mask prompts: max_i "Integrator maximum  limit:"; min_i "Integrator minimum  limit:"; i_ic "Integrator initial condition:"; max_out "Output maximum limit:"; min_out "Output minimum limit:"; Ts "Sample time: (s)"
  Product : Product  Inputs=3  SaturateOnIntegerOverflow=on  OutDataTypeStr=Inherit: Same as first input
  Relational Operator : RelationalOperator  Operator=<
  Relational Operator1 : RelationalOperator  Operator=<
  Switch : Switch  Threshold=0.5  SaturateOnIntegerOverflow=on
  Switch1 : Switch  Threshold=0.5  SaturateOnIntegerOverflow=on
  dV_ref_abc_dcvbc : Outport
  wires:
  Switch1/1 -> Product/2
  Constant1/1 -> "PI_regulator "/5(Kf), "PI_regulator "/2(Meas)
  Constant13/1 -> "PI_regulator "/3(Ki)
  Constant8/1 -> "PI_regulator "/4(Kp)
  "PI_regulator "/1(Out) -> Product/3
  Constant2/1 -> Relational Operator/2
  Constant3/1 -> Switch/1
  Constant4/1 -> Switch/3
  Relational Operator/1 -> Switch/2
  Constant5/1 -> Switch1/1
  Constant6/1 -> Switch1/3
  Relational Operator1/1 -> Switch1/2
  Switch/1 -> Product/1
  V_ref_lim_abc/1 -> Relational Operator/1
  Product/1 -> dV_ref_abc_dcvbc/1
  Iv_abc/1 -> Relational Operator1/1
  Udc_0_mean/1 -> "PI_regulator "/1(Ord)
  Constant7/1 -> Relational Operator1/2

== system HVDC_VSC_1CPUcore_dcpl/SS_HVDCStation2_WSCC2/VSC Controller (Station 2)/Discrete VSC Controller (Station 2)/Inner Current Loop/AC_Current_Control ==
  note: Uq
  note: Ud
  note: AC Current Control
  note: d axis
  note: q axis
  Iv_dq : Inport
  Iref_dq : Inport  Port=2
  U_dq : Inport  Port=3
  Freq : Inport  Port=4
  Constant1 : Constant  Value=Kp_accc
  Constant13 : Constant  Value=Ki_accc
  Constant2 : Constant  Value=1.0
  Constant3 : Constant  Value=Kf_accc
  Demux : Demux  Outputs=2
  Demux1 : Demux  Outputs=2
  Demux2 : Demux  Outputs=2
  IC: 1.0 : powerlib_extras/Discrete Measurements/Discrete Variable Frequency Mean value  Finit=50  Fmin=f_min_pll  Vinit=1.0  Ts=Ts_Control
  Mux : Mux  Inputs=2
  "PI_regulator " : Subsystem  mask(PI regulator - type 2){max_i=max_out_accc, min_i=min_out_accc, i_ic=0, max_out=max_out_accc, min_out=min_out_accc, Ts=Ts_Control}
      mask prompts: max_i "Integrator maximum  limit:"; min_i "Integrator minimum  limit:"; i_ic "Integrator initial condition:"; max_out "Output maximum limit:"; min_out "Output minimum limit:"; Ts "Sample time: (s)"
  PI_regulator_2 : Subsystem  mask(PI regulator - type 2){max_i=max_out_accc, min_i=min_out_accc, i_ic=0, max_out=max_out_accc, min_out=min_out_accc, Ts=Ts_Control}
      mask prompts: max_i "Integrator maximum  limit:"; min_i "Integrator minimum  limit:"; i_ic "Integrator initial condition:"; max_out "Output maximum limit:"; min_out "Output minimum limit:"; Ts "Sample time: (s)"
  Product : Product  SaturateOnIntegerOverflow=on  OutDataTypeStr=Inherit: Same as first input
  Product1 : Product  SaturateOnIntegerOverflow=on  OutDataTypeStr=Inherit: Same as first input
  Sum2 : Sum  Inputs=+|-|+  SaturateOnIntegerOverflow=on  InputSameDT=on  OutDataTypeStr=Inherit: Same as first input
  Sum3 : Sum  Inputs=--+  SaturateOnIntegerOverflow=on  InputSameDT=on  OutDataTypeStr=Inherit: Same as first input
  "Variable Frequency Mean value IC:1.0 " : powerlib_extras/Discrete Measurements/Discrete Variable Frequency Mean value  Finit=50  Fmin=f_min_pll  Vinit=1.0  Ts=Ts_Control
  Vref_dq_tmp : Outport
  wires:
  Constant3/1 -> Product1/1, Product/2
  Sum3/1 -> Mux/2
  IC: 1.0/1 -> Sum3/3
  Demux2/2 -> IC: 1.0/2
  Product1/1 -> Sum3/2
  Sum2/1 -> Mux/1
  "Variable Frequency Mean value IC:1.0 "/1 -> Sum2/1
  Freq/1 -> IC: 1.0/1, "Variable Frequency Mean value IC:1.0 "/1
  Demux2/1 -> "Variable Frequency Mean value IC:1.0 "/2
  Product/1 -> Sum2/3
  PI_regulator_2/1(Out) -> Sum3/1
  "PI_regulator "/1(Out) -> Sum2/2
  Iref_dq/1 -> Demux1/1
  Iv_dq/1 -> Demux/1
  Demux1/1 -> "PI_regulator "/1(Ord)  "I_ref_d"
  Demux/1 -> Product1/2, "PI_regulator "/2(Meas)  "Iv_d"
  Constant2/1 -> "PI_regulator "/5(Kf), PI_regulator_2/5(Kf)
  Demux/2 -> Product/1, PI_regulator_2/2(Meas)  "Iv_q"
  Constant13/1 -> "PI_regulator "/3(Ki), PI_regulator_2/3(Ki)
  Mux/1 -> Vref_dq_tmp/1
  Constant1/1 -> "PI_regulator "/4(Kp), PI_regulator_2/4(Kp)
  Demux1/2 -> PI_regulator_2/1(Ord)  "I_ref_q"
  U_dq/1 -> Demux2/1

== system HVDC_VSC_1CPUcore_dcpl/SS_HVDCStation2_WSCC2/VSC Controller (Station 2)/Discrete VSC Controller (Station 2)/Inner Current Loop/Inverse_Clark ==
  note: Inverse CLARK transformation
  AB0 : Inport
  Fcn1 : Fcn  Expr="1/2*(-u[1]  + sqrt(3)*u[2] + 2*u[3])"
  Fcn2 : Fcn  Expr=(u[1] - u[3])
  Fcn3 : Fcn  Expr=1/2*(-u[1] - sqrt(3)*u[2] + 2*u[3])
  Mux : Mux  Inputs=3
  abc : Outport
  wires:
  Fcn2/1 -> Mux/1
  AB0/1 -> Fcn1/1, Fcn3/1, Fcn2/1
  Fcn1/1 -> Mux/2
  Fcn3/1 -> Mux/3
  Mux/1 -> abc/1

== system HVDC_VSC_1CPUcore_dcpl/SS_HVDCStation2_WSCC2/VSC Controller (Station 2)/Discrete VSC Controller (Station 2)/Inner Current Loop/Reference_Voltage_Conditioning ==
  note: Maximum AC Voltage / DC Voltage (pole-neutral)
  note: Voltage Reference Conditioning
  Vref_dq_tmp : Inport
  Udc_meas_mean : Inport  Port=2
  Constant2 : Constant  Value=K_pwm
  Gain1 : Gain  Gain=k_pu2nom_Vdc  SaturateOnIntegerOverflow=on  OutDataTypeStr=Inherit: Same as input  ParamDataTypeStr=Inherit: Same as input
  Product1 : Product  Inputs=**/  SaturateOnIntegerOverflow=on  OutDataTypeStr=Inherit: Same as first input
  Vref_dq : Outport
  wires:
  Gain1/1 -> Product1/2
  Udc_meas_mean/1 -> Gain1/1
  Product1/1 -> Vref_dq/1
  Vref_dq_tmp/1 -> Product1/1
  Constant2/1 -> Product1/3

== system HVDC_VSC_1CPUcore_dcpl/SS_HVDCStation2_WSCC2/VSC Controller (Station 2)/Discrete VSC Controller (Station 2)/Inner Current Loop/Reference_Voltage_Limitation ==
  note: Limitation on a circle of 1 p.u. radius
  note: Reference Voltage Limitation
  note: Not Limited
  note: Limited
  Vref_dq : Inport
  Constant2 : Constant  Value=1.0
  Math Function : Math  Operator=magnitude^2  SaturateOnIntegerOverflow=on
  Math Function1 : Math  Operator=sqrt  SaturateOnIntegerOverflow=on
  Max=inf Min=eps : Saturate  UpperLimit=1e6  LowerLimit=1e-6
  Product : Product  Inputs=/*  SaturateOnIntegerOverflow=on  OutDataTypeStr=Inherit: Same as first input
  Relational Operator1 : RelationalOperator  Operator=<
  Sum : Sum  Inputs=+  SaturateOnIntegerOverflow=on
  Switch : Switch  Threshold=0.5  SaturateOnIntegerOverflow=on
  Vref_lim_dq : Outport
  wires:
  Max=inf Min=eps/1 -> Product/1
  Relational Operator1/1 -> Switch/2
  Math Function1/1 -> Max=inf Min=eps/1, Relational Operator1/1
  Vref_dq/1 -> Math Function/1, Switch/1, Product/2
  Math Function/1 -> Sum/1
  Sum/1 -> Math Function1/1
  Product/1 -> Switch/3
  Switch/1 -> Vref_lim_dq/1
  Constant2/1 -> Relational Operator1/2

== system HVDC_VSC_1CPUcore_dcpl/SS_HVDCStation2_WSCC2/VSC Controller (Station 2)/Discrete VSC Controller (Station 2)/Inner Current Loop/dq0 to abo ==
  note: X0 = X0
  note: dq0 to ab0
  note: Xa = Xd*sin(wt) + Xq*cos(wt)
  note: Xb = -Xd*cos(wt) + Xq*sin(wt)
  dq0 : Inport
  sin_cos : Inport  Port=2
  Demux : Demux  Outputs=2
  Demux1 : Demux  Outputs=3
  Mux : Mux  Inputs=3
  Product{,1..3} (4 alike) : Product  SaturateOnIntegerOverflow=on  InputSameDT=on  OutDataTypeStr=Inherit: Same as first input
  Sum1 : Sum  Inputs=+-  SaturateOnIntegerOverflow=on  InputSameDT=on  OutDataTypeStr=Inherit: Same as first input
  Sum4 : Sum  Inputs=2  SaturateOnIntegerOverflow=on  InputSameDT=on  OutDataTypeStr=Inherit: Same as first input
  ab0 : Outport
  wires:
  dq0/1 -> Demux1/1
  Mux/1 -> ab0/1
  Product3/1 -> Sum1/2
  Product2/1 -> Sum1/1
  Product1/1 -> Sum4/1
  Product/1 -> Sum4/2
  sin_cos/1 -> Demux/1
  Sum4/1 -> Mux/1
  Demux1/1 -> Product1/1, Product3/1
  Demux/1 -> Product1/2, Product2/2
  Demux/2 -> Product/2, Product3/2
  Demux1/2 -> Product/1, Product2/1
  Sum1/1 -> Mux/2
  Demux1/3 -> Mux/3
